simulink model "SimMRT"  (R2023b)
settings: Solver=VariableStepAuto  StartTime=0.0  StopTime=10.0  RelTol=1e-3

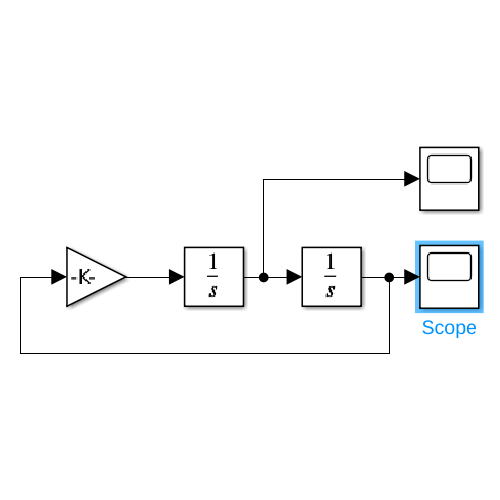
[thumbnail: Simulink's stored preview of the top-level diagram]
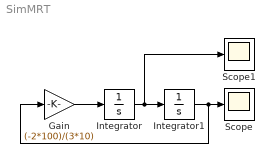
== system SimMRT ==
  Gain : Gain  Gain=(-2*100)/(3*10)
  Integrator : Integrator  InitialCondition=2
  Integrator1 : Integrator
  Scope : Scope
  Scope1 : Scope
  wires:
  Integrator/1 -> Scope1/1, Integrator1/1
  Gain/1 -> Integrator/1
  Integrator1/1 -> Gain/1, Scope/1
